simulink model "minFullSim"  (R2015b)
settings: Solver=VariableStepAuto  StartTime=0.0  StopTime=1  RelTol=1e-3
settings Model: Creator=Ricardo  LastModifiedBy=Ricardo

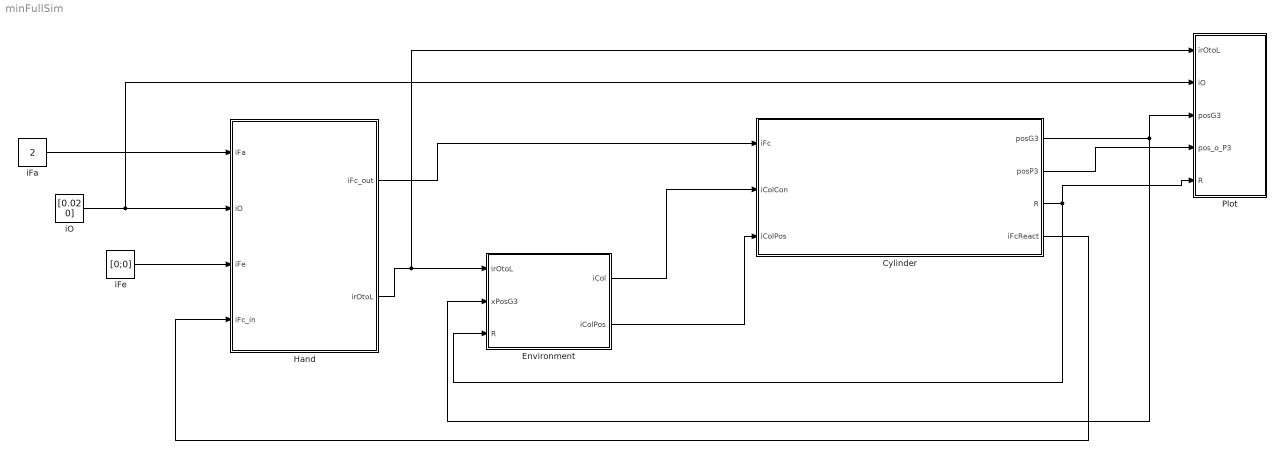
== system minFullSim ==
  Cylinder : Subsystem
  Environment : Subsystem
  Hand : Subsystem
  Plot : Subsystem
  iFa : Constant  Value=2
  iFe : Constant  Value=[0;0]
  iO : Constant  Value=[0.02 0]
  wires:
  Hand/2(irOtoL) -> Plot/1(irOtoL), Environment/1(irOtoL)
  Environment/1(iCol) -> Cylinder/2(iColCon)
  Environment/2(iColPos) -> Cylinder/3(iColPos)
  Hand/1(iFc_out) -> Cylinder/1(iFc)
  iFa/1 -> Hand/1(iFa)
  iO/1 -> Plot/2(iO), Hand/2(iO)
  iFe/1 -> Hand/3(iFe)
  Cylinder/3(R) -> Plot/5(R), Environment/3(R)
  Cylinder/4(iFcReact) -> Hand/4(iFc_in)
  Cylinder/2(posP3) -> Plot/4(pos_o_P3)
  Cylinder/1(posG3) -> Plot/3(posG3), Environment/2(xPosG3)

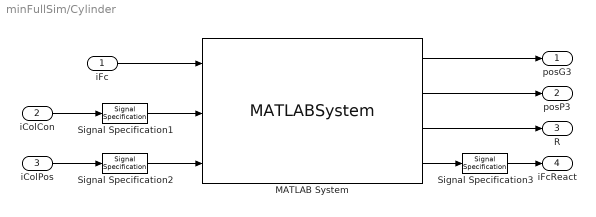
== system minFullSim/Cylinder ==
  iFc : Inport
  iColCon : Inport  Port=2
  iColPos : Inport  Port=3
  MATLAB System : MATLABSystem  System=MinCylinderTester  R=0.02  M=0.003  g=9.81  Us=0.5  Uk=0.48  Urs=0.5  Urk=0.48  Ucs=0.5  Uck=0.4  Iz=6e-07  F_s_x=0.014715  F_s_y=0.014715  F_k_x=0.0141264  F_k_y=0.0141264  T_s=0.0001962  T_k=0.000188352  Position_o_G3=[0;0.16]  Position_G3_P3_frame_cylinder=[ 0; 0.02]  SimulateUsing=Interpreted execution
      mask Type: MinCylinderTester
      mask Display:
      | disp('MinCylinderTester');
      | port_label('input',1,'IndexFext');
      | port_label('input',2,'CollisionCondition');
      | port_label('input',3,'CollisionPosition');
      | port_label('output',1,'PositionO_G3');
      | port_label('output',2,'PositionO_P3');
      | port_label('output',3,'Radius');
      | port_label('output',4,'ForceReactionIndex');
  Signal Specification1 : SignalSpecification  Dimensions=1
  Signal Specification2 : SignalSpecification  Dimensions=2
  Signal Specification3 : SignalSpecification  Dimensions=[2 1]
  posG3 : Outport
  posP3 : Outport  Port=2
  R : Outport  Port=3
  iFcReact : Outport  Port=4
  wires:
  iFc/1 -> MATLAB System/1
  MATLAB System/1 -> posG3/1
  MATLAB System/2 -> posP3/1
  MATLAB System/3 -> R/1
  iColCon/1 -> Signal Specification1/1
  iColPos/1 -> Signal Specification2/1
  Signal Specification1/1 -> MATLAB System/2
  Signal Specification2/1 -> MATLAB System/3
  Signal Specification3/1 -> iFcReact/1
  MATLAB System/4 -> Signal Specification3/1

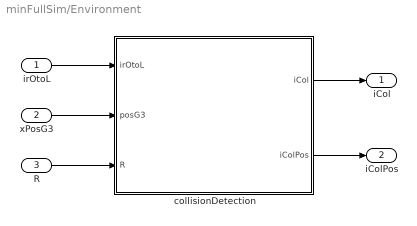
== system minFullSim/Environment ==
  irOtoL : Inport
  xPosG3 : Inport  Port=2
  R : Inport  Port=3
  collisionDetection : MATLAB Function  TreatAsAtomicUnit=on
  iCol : Outport
  iColPos : Outport  Port=2
  wires:
  irOtoL/1 -> collisionDetection/1(irOtoL)
  xPosG3/1 -> collisionDetection/2(posG3)
  collisionDetection/1(iCol) -> iCol/1
  collisionDetection/2(iColPos) -> iColPos/1
  R/1 -> collisionDetection/3(R)

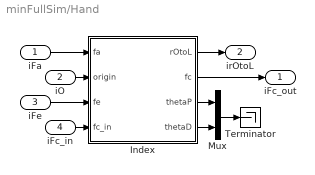
== system minFullSim/Hand ==
  iFa : Inport
  iO : Inport  Port=2
  iFe : Inport  Port=3
  iFc_in : Inport  Port=4
  Index : Subsystem
  Mux : Mux  Inputs=2
  Terminator : Terminator
  iFc_out : Outport
  irOtoL : Outport  Port=2
  wires:
  iO/1 -> Index/2(origin)
  iFe/1 -> Index/3(fe)
  iFc_in/1 -> Index/4(fc_in)
  Index/1(rOtoL) -> irOtoL/1
  Index/2(fc) -> iFc_out/1
  Index/3(thetaP) -> Mux/1
  Index/4(thetaD) -> Mux/2
  iFa/1 -> Index/1(fa)
  Mux/1 -> Terminator/1

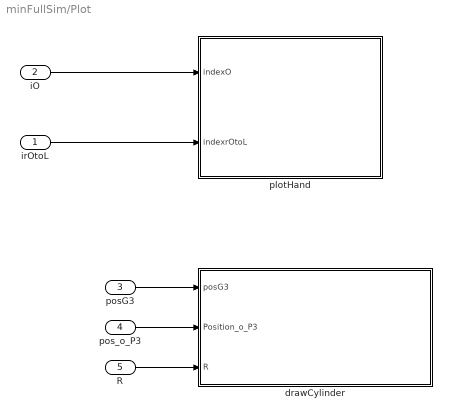
== system minFullSim/Plot ==
  irOtoL : Inport
  iO : Inport  Port=2
  posG3 : Inport  Port=3
  pos_o_P3 : Inport  Port=4
  R : Inport  Port=5
  drawCylinder : MATLAB Function  TreatAsAtomicUnit=on
  plotHand : MATLAB Function  TreatAsAtomicUnit=on
  wires:
  iO/1 -> plotHand/1(indexO)
  irOtoL/1 -> plotHand/2(indexrOtoL)
  posG3/1 -> drawCylinder/1(posG3)
  pos_o_P3/1 -> drawCylinder/2(Position_o_P3)
  R/1 -> drawCylinder/3(R)

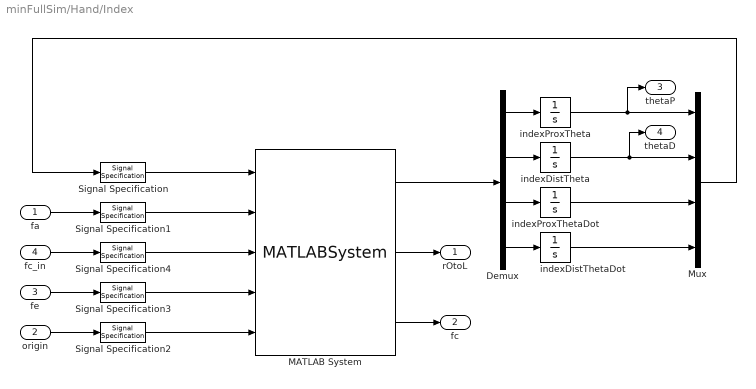
== system minFullSim/Hand/Index ==
  fa : Inport
  origin : Inport  Port=2
  fe : Inport  Port=3
  fc_in : Inport  Port=4
  Demux : Demux
  MATLAB System : MATLABSystem  System=Index  kP=-0.043  kD=-0.185  dP=-0.01  dD=-0.01  lP=0.1  lD=0.1  rP=0.02  rD=0.012  mP=0.02  mD=0.02  thetaP=pi/10  thetaD=pi/3  SimulateUsing=Interpreted execution
      mask Type: Index
      mask Display:
      | disp('Index');
      | port_label('input',1,'initVal');
      | port_label('input',2,'fa');
      | port_label('input',3,'fc');
      | port_label('input',4,'fe');
      | port_label('input',5,'origin');
      | port_label('output',1,'xDot');
      | port_label('output',2,'rOtoL');
      | port_label('output',3,'fc');
  Mux : Mux
  Signal Specification : SignalSpecification  Dimensions=4
  Signal Specification1 : SignalSpecification  Dimensions=1
  Signal Specification2 : SignalSpecification  Dimensions=2
  Signal Specification3 : SignalSpecification  Dimensions=2
  Signal Specification4 : SignalSpecification  Dimensions=2
  indexDistTheta : Integrator  InitialCondition=pi/3  ContinuousStateAttributes='indexDistTheta'
  indexDistThetaDot : Integrator  ContinuousStateAttributes='indexDistThetaDot'
  indexProxTheta : Integrator  InitialCondition=pi/10  ContinuousStateAttributes='indexProxTheta'
  indexProxThetaDot : Integrator  ContinuousStateAttributes='indexProxThetaDot'
  rOtoL : Outport
  fc : Outport  Port=2
  thetaP : Outport  Port=3
  thetaD : Outport  Port=4
  wires:
  Demux/1 -> indexProxTheta/1
  Demux/2 -> indexDistTheta/1
  Demux/3 -> indexProxThetaDot/1
  Demux/4 -> indexDistThetaDot/1
  MATLAB System/1 -> Demux/1
  indexProxTheta/1 -> Mux/1, thetaP/1
  indexDistTheta/1 -> Mux/2, thetaD/1
  indexProxThetaDot/1 -> Mux/3
  indexDistThetaDot/1 -> Mux/4
  Mux/1 -> Signal Specification/1
  Signal Specification/1 -> MATLAB System/1
  MATLAB System/2 -> rOtoL/1
  MATLAB System/3 -> fc/1
  Signal Specification1/1 -> MATLAB System/2
  fa/1 -> Signal Specification1/1
  origin/1 -> Signal Specification2/1
  Signal Specification2/1 -> MATLAB System/5
  fe/1 -> Signal Specification3/1
  Signal Specification3/1 -> MATLAB System/4
  fc_in/1 -> Signal Specification4/1
  Signal Specification4/1 -> MATLAB System/3

== matlab function minFullSim/Environment/collisionDetection ==
  data: irOtoL input; iCol output; posG3 input; R input; iColPos output
% Handles collision detection between fingertips and Cylinder. 
% Handled in Simulink.
% Author: Ricardo Garcia Rosas
% Change log:
%%%%%%%%%%%%|%%%%%%%%%%%|%%%%%%%%%%%%%%%%%%%%%%%%%%%%%%%%%%%%%%%%%%%|
% Date      |   Author  | Notes                                     |
% 16/04/06  |   RGR     | Created.                                  |
function [iCol,iColPos] = collisionDetection(irOtoL,posG3,R)
    % Handles collision detection between fingertips and Cylinder.
    % Performed by comparing object radius.
    iCol = false;
    iColPos = [0;0];
    % Get circle radius given object center and fingertip position.
    ri = sqrt((irOtoL(1,2)-posG3(1,1))^2+(irOtoL(2,2)-posG3(2,1))^2);
    % Verify calculated radius with object radius to define collision.
    if(ri<=R)
        iCol = true;
        iColPos = irOtoL(:,2);
    else
        iCol = false;
        iColPos = [0;0];
    end    
end

== matlab function minFullSim/Plot/plotHand ==
  data: indexO input; indexrOtoL input
% Plots the entire hand to the default figure. Handled in Simulink.
% Author: Ricardo Garcia Rosas
% Change log:
%%%%%%%%%%%%|%%%%%%%%%%%|%%%%%%%%%%%%%%%%%%%%%%%%%%%%%%%%%%%%%%%%%%%|
% Date      |   Author  | Notes                                     |
% 16/03/23  |   RGR     | Added more comments.                      |
function plotHand(indexO,indexrOtoL)
    % Plots the entire hand to the default figure. Handled in Simulink.
    % @param indexO Index finger origin position [x,y] (m).
    % @param indexrOtoL Index finger vector from its origin to its link
    % ends.
    % @param thumbO Thumb origin position [x,y] (m).
    % @param thumbrOtoL Thumb vector from its origin to its link ends.

    % Call figure
    figure(1);
    clf;
    hold on;
    % Draw pam
    plot([indexO(1) thumbO(1)],[indexO(2) thumbO(2)],'LineWidth',8,'Color', 'k');
    % Draw Proximal components of Index
    plot([indexO(1) indexrOtoL(1,1)],[indexO(2) indexrOtoL(2,1)],'LineWidth',8,'Color', 'k');
    plot(indexO(1),indexO(2),'ko','MarkerSize',18);
    % Draw Distal components of Index
    plot([indexrOtoL(1,1) indexrOtoL(1,2)],[indexrOtoL(2,1) indexrOtoL(2,2)],'LineWidth',8,'Color', 'k');
    plot(indexrOtoL(1,1),indexrOtoL(2,1),'ko','MarkerSize',18);
    % Draw Index fingertip
    plot(indexrOtoL(1,2),indexrOtoL(2,2),'ko','MarkerSize',8);
    hold off;
    axis([-0.2 0.2 -0.05 0.2]);
end

== matlab function minFullSim/Plot/drawCylinder ==
  data: posG3 input; Position_o_P3 input; R input
function DrawCylinder(posG3,Position_o_P3,R)
%#
    figure(1);
    hold on
    t=linspace(0,2*pi,360);
    plot(posG3(1,1),posG3(2,1),'r*');
    plot(Position_o_P3(1),Position_o_P3(2),'r*');
    x=posG3(1,1)+R*cos(t);
    y=posG3(2,1)+R*sin(t);
    plot(x,y,'b');
    hold off
    axis([-0.2 0.2 -0.05 0.2]);
end
